simulink model "sistemaLazoAbiertoLineal_con_transfPark2017"  (R2017a)
settings: Solver=ode45  StartTime=0.0  StopTime=5  MaxStep=0.0001  RelTol=1e-3  EnableMultiTasking=on
values from neighbouring files (symbols this model uses):
  alfa_cu = 3.9*10^-3    (= 0.0039)    [InicializaYconstantes.m]
  b_m = bm+(bl/r^2)    (= 1.5e-05)    [InicializaYconstantes.m]
  Cts = 1.091    [InicializaYconstantes.m]
  J_m = Jm+(Jl/r^2)    (= 5.65099476805e-06)    [InicializaYconstantes.m]
  lambda = 0.01546    [InicializaYconstantes.m]
  Ld = 6.6*10^-3    (= 0.0066)    [InicializaYconstantes.m]
  Lq = 5.8*10^-3    (= 0.0058)    [InicializaYconstantes.m]
  Pp = 3    [InicializaYconstantes.m]
  Rs = 1.02    [InicializaYconstantes.m]
  Rs_cero = 1.02    [InicializaYconstantes.m]
  Rts = 55    [InicializaYconstantes.m]
  T_l = Tl/r    (= 0.00499521477515)    [InicializaYconstantes.m]
  Ta = 40    [InicializaYconstantes.m]
  Ts0 = 40    [InicializaYconstantes.m]
settings Model: Creator=usuario  LastModifiedBy=usuario
settings DataIOCC: LimitDataPoints=on  SaveFormat=Array
settings OptimizationCC: ExpressionDepthLimit=2147483647  LifeSpan=inf
settings DebuggingCC: UnderspecifiedInitializationDetection=Classic  MergeDetectMultiDrivingBlocksExec=none  SolverPrmCheckMsg=warning  StateNameClashWarn=warning  SFUnexpectedBacktrackingDiag=warning  SFNoUnconditionalDefaultTransitionDiag=warning  SFExecutionAtInitializationDiag=none
settings HardwareCC: ProdBitPerPointer=32  ProdBitPerSizeT=32  ProdBitPerPtrDiffT=32  ProdLargestAtomicFloat=None  ProdIntDivRoundTo=Undefined  ProdEndianess=Unspecified  ProdWordSize=32  ProdHWDeviceType=32-bit Generic
settings ModelReferenceCC: PropagateSignalLabelsOutOfModel=off
settings GRTTargetCC: TargetLangStandard=C89/C90 (ANSI)  GeneratePreprocessorConditionals=Disable all
settings ConfigComp: CovMetricSettings=dw  CovHtmlReporting=on  CovSaveCumulativeToWorkspaceVar=on  CovSaveSingleToWorkspaceVar=on  CovExternalEMLEnable=off

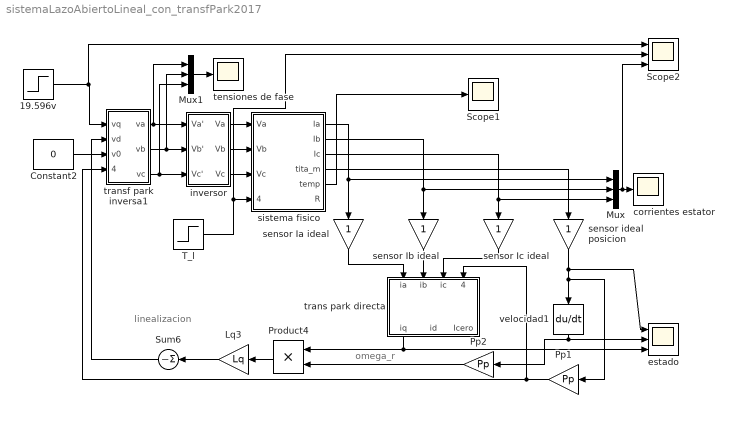
== system sistemaLazoAbiertoLineal_con_transfPark2017 ==
  note: omega_r
  note: linealizacion
  19.596v : Step  Time=0.1  After=19.596  SampleTime=0
  Constant2 : Constant  Value=0
  Lq3 : Gain  Gain=Lq
  Mux : Mux  Inputs=3
  Mux1 : Mux  Inputs=3
  Pp1 : Gain  Gain=Pp
  Pp2 : Gain  Gain=Pp
  Product4 : Product  RndMeth=Zero
  Scope1 : Scope
  Scope2 : Scope  NumInputPorts=3
  Sum6 : Sum  Inputs=-
  T_l : Step  Time=0.3  After=T_l  SampleTime=0
  corrientes estator : Scope
  estado : Scope  NumInputPorts=3
  inversor : Subsystem
  sensor ideal posicion : Gain
  sensor Ia ideal : Gain
  sensor Ib ideal : Gain
  sensor Ic ideal : Gain
  sistema fisico : Subsystem
  tensiones de fase : Scope
  trans park directa : Subsystem
  transf park inversa1 : Subsystem
  velocidad1 : Derivative
  wires:
  19.596v/1 -> Scope2/1, transf park inversa1/1(vq)
  Constant2/1 -> transf park inversa1/3(v0)
  velocidad1/1 -> estado/2, Pp2/1
  sistema fisico/1(Ia) -> sensor Ia ideal/1, Mux/1
  sensor Ia ideal/1 -> trans park directa/1(ia)
  sensor Ib ideal/1 -> trans park directa/2(ib)
  sensor Ic ideal/1 -> trans park directa/3(ic)
  trans park directa/1(iq) -> estado/3, Product4/1
  Product4/1 -> Lq3/1
  Lq3/1 -> Sum6/1
  Sum6/1 -> transf park inversa1/2(vd)
  inversor/1(Va) -> sistema fisico/1(Va)
  inversor/2(Vb) -> sistema fisico/2(Vb)
  inversor/3(Vc) -> sistema fisico/3(Vc)
  sistema fisico/2(Ib) -> sensor Ib ideal/1, Mux/2
  sistema fisico/3(Ic) -> sensor Ic ideal/1, Mux/3
  Mux/1 -> Scope2/3, corrientes estator/1
  transf park inversa1/3(vc) -> Mux1/3, inversor/3(Vc')
  transf park inversa1/2(vb) -> Mux1/2, inversor/2(Vb')
  transf park inversa1/1(va) -> Mux1/1, inversor/1(Va')
  sistema fisico/4(tita_m) -> sensor ideal posicion/1
  sensor ideal posicion/1 -> Pp1/1, velocidad1/1, estado/1
  T_l/1 -> Scope2/2, sistema fisico/4(perturbacion)
  Mux1/1 -> tensiones de fase/1
  Pp1/1 -> transf park inversa1/4(tita_r), trans park directa/4(tita_r)
  sistema fisico/5(temp) -> Scope1/1
  Pp2/1 -> Product4/2

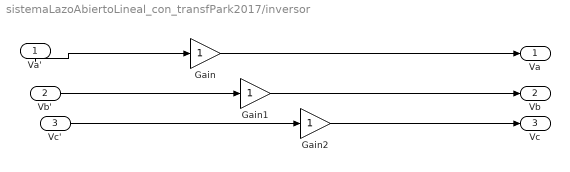
== system sistemaLazoAbiertoLineal_con_transfPark2017/inversor ==
  Va' : Inport
  Vb' : Inport  Port=2
  Vc' : Inport  Port=3
  Gain : Gain
  Gain1 : Gain
  Gain2 : Gain
  Va : Outport
  Vb : Outport  Port=2
  Vc : Outport  Port=3
  wires:
  Gain/1 -> Va/1
  Gain1/1 -> Vb/1
  Vb'/1 -> Gain1/1
  Va'/1 -> Gain/1
  Vc'/1 -> Gain2/1
  Gain2/1 -> Vc/1

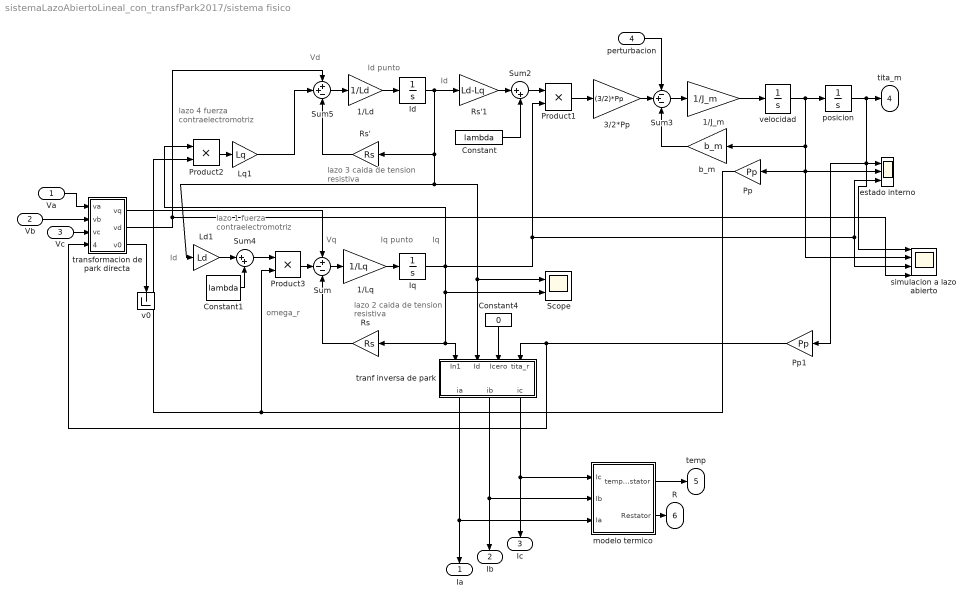
== system sistemaLazoAbiertoLineal_con_transfPark2017/sistema fisico ==
  note: Id
  note: lazo 4 fuerza
      |  contraelectromotriz
  note: lazo 3 caida de
      |  tension resistiva
  note: lazo 2 caida de
      |  tension resistiva
  note: lazo 1 fuerza
      |  contraelectromotriz
  note: Vd
  note: Iq
  note: Id punto
  note: Vq
  note: Iq punto
  note: Id
  note: omega_r
  Va : Inport
  Vb : Inport  Port=2
  Vc : Inport  Port=3
  perturbacion : Inport  Port=4
  1/J_m : Gain  Gain=1/J_m
  1/Ld : Gain  Gain=1/Ld
  1/Lq : Gain  Gain=1/Lq
  3/2*Pp : Gain  Gain=(3/2)*Pp
  Constant : Constant  Value=lambda
  Constant1 : Constant  Value=lambda
  Constant4 : Constant  Value=0
  Id : Integrator
  Iq : Integrator
  Ld1 : Gain  Gain=Ld
  Lq1 : Gain  Gain=Lq
  Pp : Gain  Gain=Pp
  Pp1 : Gain  Gain=Pp
  Product1 : Product  RndMeth=Zero
  Product2 : Product  RndMeth=Zero
  Product3 : Product  RndMeth=Zero
  Rs : Gain  Gain=Rs
  Rs' : Gain  Gain=Rs
  Rs'1 : Gain  Gain=Ld-Lq
  Scope : Scope  NumInputPorts=2
  Sum : Sum  Inputs=+--
  Sum2 : Sum  Inputs=|++
  Sum3 : Sum  Inputs=-+-
  Sum4 : Sum  Inputs=|++
  Sum5 : Sum  Inputs=++-
  b_m : Gain  Gain=b_m
  estado interno : Scope  NumInputPorts=3
  modelo termico : Subsystem
  posicion : Integrator
  simulacion a lazo abierto : Scope  NumInputPorts=4
  "tranf inversa de park " : Subsystem
  transformacion de park directa : Subsystem
  v0 : Terminator
  velocidad : Integrator  ContinuousStateAttributes='velocidad'
  Ia : Outport
  Ib : Outport  Port=2
  Ic : Outport  Port=3
  tita_m : Outport  Port=4
  temp : Outport  Port=5
  R : Outport  Port=6
  wires:
  Constant/1 -> Sum2/2
  Sum2/1 -> Product1/1
  1/Lq/1 -> Iq/1
  Product1/1 -> 3/2*Pp/1
  Ld1/1 -> Sum4/1
  Sum3/1 -> 1/J_m/1
  1/Ld/1 -> Id/1
  Constant1/1 -> Sum4/2
  b_m/1 -> Sum3/3
  Sum/1 -> 1/Lq/1
  Rs/1 -> Sum/3
  perturbacion/1 -> Sum3/1
  Rs'/1 -> Sum5/3
  Product2/1 -> Lq1/1
  Iq/1 -> Scope/2, Rs/1, "tranf inversa de park "/1(In1), Product2/1, Product1/2, simulacion a lazo abierto/3, estado interno/3
  Product3/1 -> Sum/2
  transformacion de park directa/1(vq) -> Sum/1
  transformacion de park directa/2(vd) -> simulacion a lazo abierto/4, Sum5/1
  Sum5/1 -> 1/Ld/1
  3/2*Pp/1 -> Sum3/2
  1/J_m/1 -> velocidad/1
  Lq1/1 -> Sum5/2
  transformacion de park directa/3(v0) -> v0/1
  Sum4/1 -> Product3/1
  Id/1 -> Rs'1/1, Rs'/1, Scope/1, "tranf inversa de park "/2(Id), Ld1/1
  Constant4/1 -> "tranf inversa de park "/3(Icero)
  Vc/1 -> transformacion de park directa/3(vc)
  Vb/1 -> transformacion de park directa/2(vb)
  Va/1 -> transformacion de park directa/1(va)
  "tranf inversa de park "/1(ia) -> modelo termico/3(Ia), Ia/1
  "tranf inversa de park "/2(ib) -> modelo termico/2(Ib), Ib/1
  "tranf inversa de park "/3(ic) -> modelo termico/1(Ic), Ic/1
  velocidad/1 -> posicion/1, simulacion a lazo abierto/2, estado interno/2, Pp/1, b_m/1
  modelo termico/1(tempEstator) -> temp/1
  modelo termico/2(Restator) -> R/1
  Pp/1 -> Product2/2, Product3/2
  posicion/1 -> tita_m/1, simulacion a lazo abierto/1, Pp1/1, estado interno/1
  Rs'1/1 -> Sum2/1
  Pp1/1 -> transformacion de park directa/4(tita_r), "tranf inversa de park "/4(tita_r)

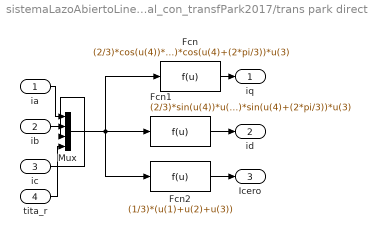
== system sistemaLazoAbiertoLineal_con_transfPark2017/trans park directa ==
  ia : Inport
  ib : Inport  Port=2
  ic : Inport  Port=3
  tita_r : Inport  Port=4
  Fcn : Fcn  Expr=(2/3)*cos(u(4))*u(1)+(2/3)*cos(u(4)-(2*pi/3))*u(2)+(2/3)*cos(u(4)+(2*pi/3))*u(3)
  Fcn1 : Fcn  Expr=(2/3)*sin(u(4))*u(1)+(2/3)*sin(u(4)-(2*pi/3))*u(2)+(2/3)*sin(u(4)+(2*pi/3))*u(3)
  Fcn2 : Fcn  Expr=(1/3)*(u(1)+u(2)+u(3))
  Mux : Mux
  iq : Outport
  id : Outport  Port=2
  Icero : Outport  Port=3
  wires:
  Mux/1 -> Fcn1/1, Fcn/1, Fcn2/1
  Fcn/1 -> iq/1
  ia/1 -> Mux/1
  ib/1 -> Mux/2
  Fcn1/1 -> id/1
  ic/1 -> Mux/3
  tita_r/1 -> Mux/4
  Fcn2/1 -> Icero/1

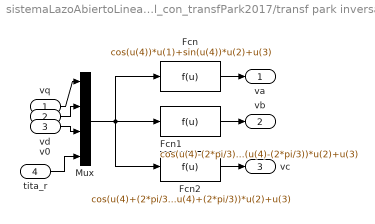
== system sistemaLazoAbiertoLineal_con_transfPark2017/transf park inversa1 ==
  vq : Inport
  vd : Inport  Port=2
  v0 : Inport  Port=3
  tita_r : Inport  Port=4
  Fcn : Fcn  Expr=cos(u(4))*u(1)+sin(u(4))*u(2)+u(3)
  Fcn1 : Fcn  Expr=cos(u(4)-(2*pi/3))*u(1)+sin(u(4)-(2*pi/3))*u(2)+u(3)
  Fcn2 : Fcn  Expr=cos(u(4)+(2*pi/3))*u(1)+sin(u(4)+(2*pi/3))*u(2)+u(3)
  Mux : Mux
  va : Outport
  vb : Outport  Port=2
  vc : Outport  Port=3
  wires:
  Mux/1 -> Fcn2/1, Fcn1/1, Fcn/1
  Fcn/1 -> va/1
  vq/1 -> Mux/1
  vd/1 -> Mux/2
  Fcn1/1 -> vb/1
  v0/1 -> Mux/3
  tita_r/1 -> Mux/4
  Fcn2/1 -> vc/1

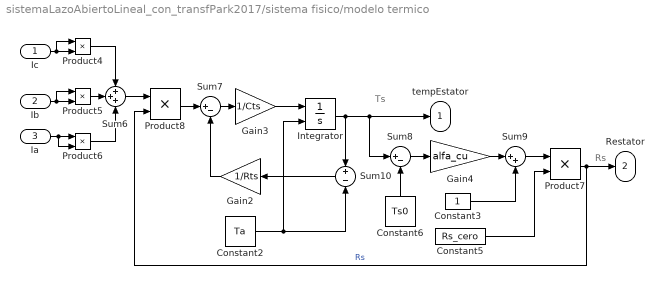
== system sistemaLazoAbiertoLineal_con_transfPark2017/sistema fisico/modelo termico ==
  note: Ts
  note: Rs
  Ic : Inport
  Ib : Inport  Port=2
  Ia : Inport  Port=3
  Constant2 : Constant  Value=Ta
  Constant3 : Constant
  Constant5 : Constant  Value=Rs_cero
  Constant6 : Constant  Value=Ts0
  Gain2 : Gain  Gain=1/Rts
  Gain3 : Gain  Gain=1/Cts
  Gain4 : Gain  Gain=alfa_cu
  Integrator : Integrator  InitialConditionSource=external
  Product{4..8} (5 alike) : Product  RndMeth=Zero
  Sum10 : Sum  Inputs=+-
  Sum6 : Sum  Inputs=+++
  Sum7 : Sum  Inputs=|+-
  Sum8 : Sum  Inputs=|+-
  Sum9 : Sum  Inputs=|++
  tempEstator : Outport
  Restator : Outport  Port=2
  wires:
  Gain2/1 -> Sum7/2
  Product4/1 -> Sum6/1
  Gain4/1 -> Sum9/1
  Product6/1 -> Sum6/3
  Gain3/1 -> Integrator/1
  Sum7/1 -> Gain3/1
  Product7/1 -> Product8/2, Restator/1  "Rs"
  Integrator/1 -> Sum10/1, Sum8/1, tempEstator/1
  Constant5/1 -> Product7/2
  Sum9/1 -> Product7/1
  Sum8/1 -> Gain4/1
  Constant3/1 -> Sum9/2
  Sum6/1 -> Product8/1
  Product5/1 -> Sum6/2
  Constant6/1 -> Sum8/2
  Constant2/1 -> Integrator/2, Sum10/2
  Product8/1 -> Sum7/1
  Sum10/1 -> Gain2/1
  Ib/1 -> Product5/1, Product5/2
  Ia/1 -> Product6/2, Product6/1
  Ic/1 -> Product4/1, Product4/2

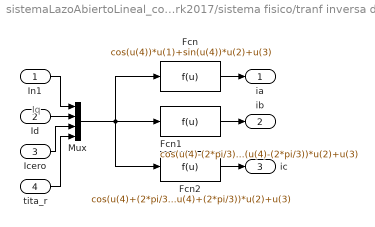
== system sistemaLazoAbiertoLineal_con_transfPark2017/sistema fisico/tranf inversa de park  ==
  note: Iq
  In1 : Inport
  Id : Inport  Port=2
  Icero : Inport  Port=3
  tita_r : Inport  Port=4
  Fcn : Fcn  Expr=cos(u(4))*u(1)+sin(u(4))*u(2)+u(3)
  Fcn1 : Fcn  Expr=cos(u(4)-(2*pi/3))*u(1)+sin(u(4)-(2*pi/3))*u(2)+u(3)
  Fcn2 : Fcn  Expr=cos(u(4)+(2*pi/3))*u(1)+sin(u(4)+(2*pi/3))*u(2)+u(3)
  Mux : Mux
  ia : Outport
  ib : Outport  Port=2
  ic : Outport  Port=3
  wires:
  Mux/1 -> Fcn1/1, Fcn/1, Fcn2/1
  Fcn/1 -> ia/1
  In1/1 -> Mux/1
  Id/1 -> Mux/2
  Fcn1/1 -> ib/1
  Icero/1 -> Mux/3
  tita_r/1 -> Mux/4
  Fcn2/1 -> ic/1

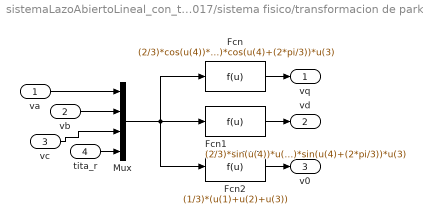
== system sistemaLazoAbiertoLineal_con_transfPark2017/sistema fisico/transformacion de park directa ==
  va : Inport
  vb : Inport  Port=2
  vc : Inport  Port=3
  tita_r : Inport  Port=4
  Fcn : Fcn  Expr=(2/3)*cos(u(4))*u(1)+(2/3)*cos(u(4)-(2*pi/3))*u(2)+(2/3)*cos(u(4)+(2*pi/3))*u(3)
  Fcn1 : Fcn  Expr=(2/3)*sin(u(4))*u(1)+(2/3)*sin(u(4)-(2*pi/3))*u(2)+(2/3)*sin(u(4)+(2*pi/3))*u(3)
  Fcn2 : Fcn  Expr=(1/3)*(u(1)+u(2)+u(3))
  Mux : Mux
  vq : Outport
  vd : Outport  Port=2
  v0 : Outport  Port=3
  wires:
  Mux/1 -> Fcn2/1, Fcn1/1, Fcn/1
  Fcn/1 -> vq/1
  va/1 -> Mux/1
  vb/1 -> Mux/2
  Fcn1/1 -> vd/1
  vc/1 -> Mux/3
  tita_r/1 -> Mux/4
  Fcn2/1 -> v0/1
